simulink model "atividade1_Simulacao"  (Simulink 7.1)
settings: Solver=ode45  StartTime=0.0  StopTime=10  RelTol=1e-3
settings Model: Creator=CARLOS BRUNO  LastModifiedBy=CARLOS BRUNO

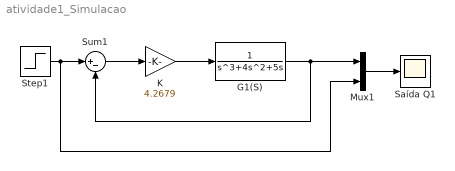
== system atividade1_Simulacao ==
  G1(S) : TransferFcn  Denominator=[1 4 5 0]
  K : Gain  Gain=4.2679  ParameterDataType=sfix(16)  ParameterScaling=2^0  OutDataType=sfix(16)  OutScaling=2^0
  Mux1 : Mux  Inputs=2
  Saída Q1 : Scope
      settings: TimeRange=20  YMin=5.55112e-017  YMax=1
  Step1 : Step  Time=0  SampleTime=0
  Sum1 : Sum  Inputs=|+-  OutDataType=sfix(16)  OutScaling=2^0
  wires:
  Step1/1 -> Sum1/1, Mux1/2
  Mux1/1 -> Saída Q1/1
  G1(S)/1 -> Mux1/1, Sum1/2
  Sum1/1 -> K/1
  K/1 -> G1(S)/1
